simulink model "sim2"  (R2022a)
settings: Solver=VariableStepAuto  StartTime=0.0  StopTime=10.0  RelTol=1e-3
undefined symbols (not defined in the file or in its folder): pointX, pointY
libraries: robotcorelib x1
settings Model: Creator=loryb  LastModifiedBy=loryb

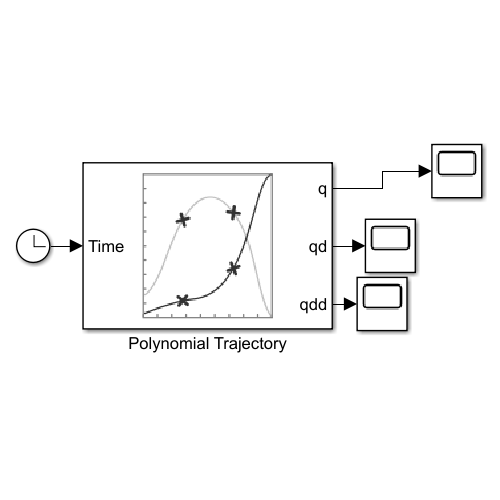
[thumbnail: Simulink's stored preview of the top-level diagram]
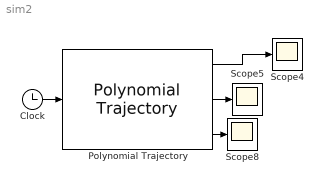
== system sim2 ==
  Clock : Clock
  Polynomial Trajectory : robotcorelib/Polynomial Trajectory  WaypointSource=Internal  Waypoints=[pointX;pointY]  TimePoints=sampletime  TimeInterval=[ 1, 4 ]  Method=Quintic Polynomial  ParameterSource=Internal  VelocityBoundaryCondition=velBound'  AccelerationBoundaryCondition=aBound'  SimulateUsing=Interpreted execution
      settings: SourceProductBaseCode=RO,NV,RR,UV
  Scope4 : Scope
  Scope5 : Scope
  Scope8 : Scope
  wires:
  Clock/1 -> Polynomial Trajectory/1
  Polynomial Trajectory/2 -> Scope5/1
  Polynomial Trajectory/1 -> Scope4/1
  Polynomial Trajectory/3 -> Scope8/1
